simulink model "peto"  (R2017b)
settings: Solver=VariableStepAuto  StartTime=0.0  StopTime=5.0  RelTol=1e-3
undefined symbols (not defined in the file): a, b, p, q, x0, y0
settings Model: Creator=Timo Järvinen  LastModifiedBy=Timo Järvinen

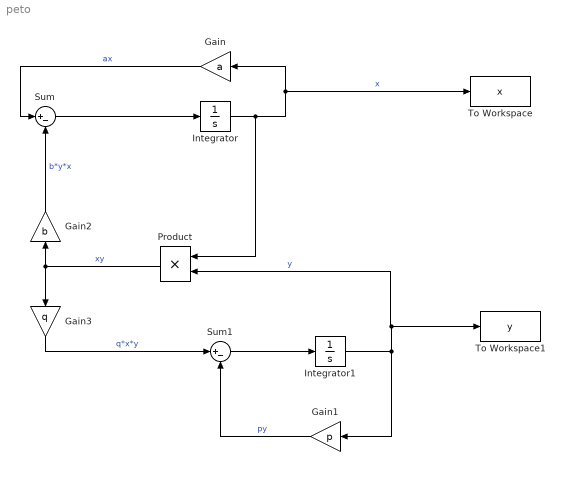
== system peto ==
  Gain : Gain  Gain=a
  Gain1 : Gain  Gain=p
  Gain2 : Gain  Gain=b
  Gain3 : Gain  Gain=q
  Integrator : Integrator  InitialCondition=x0
  Integrator1 : Integrator  InitialCondition=y0
  Product : Product
  Sum : Sum  Inputs=|+-
  Sum1 : Sum  Inputs=|+-
  To Workspace : ToWorkspace  VariableName=x  SampleTime=-1
  To Workspace1 : ToWorkspace  VariableName=y  SampleTime=-1
  wires:
  Integrator/1 -> Product/1, Gain/1, To Workspace/1  "x"
  Sum/1 -> Integrator/1
  Gain/1 -> Sum/1  "ax"
  Integrator1/1 -> Product/2, To Workspace1/1, Gain1/1  "y"
  Gain2/1 -> Sum/2  "b*y*x"
  Sum1/1 -> Integrator1/1
  Gain1/1 -> Sum1/2  "py"
  Product/1 -> Gain3/1, Gain2/1  "xy"
  Gain3/1 -> Sum1/1  "q*x*y"
